simulink model "semifinal"  (R2020a)
settings: Solver=VariableStepAuto  StartTime=0.0  StopTime=50.0  RelTol=1e-3
undefined symbols (not defined in the file): D1, Delta
libraries: powerlib x39, sps_avr x2
settings Model: Creator=USER  LastModifiedBy=USER

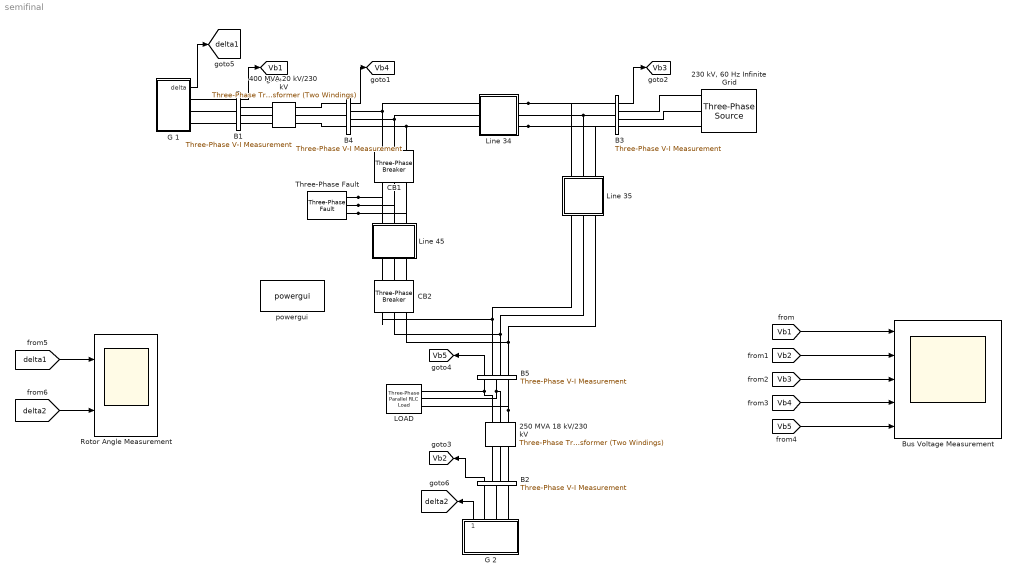
== system semifinal ==
  "    Line 35 " : Subsystem
  "230 kV, 60 Hz Infinite Grid" : powerlib/Electrical Sources/Three-Phase Source  InternalConnection=Yg  VoltagePhases=off  Voltage=230e3  PhaseAngle=0  Voltage_phases=[25e3 25e3 25e3]/sqrt(3)  PhaseAngles_phases=[0 -120 +120]  Frequency=60  NonIdealSource=on  SpecifyImpedance=off  Resistance=0.00000000000000001  Inductance=16.58e-3  ShortCircuitLevel=100e6  BaseVoltage=230e3  XRratio=7  BusType=swing  Pref=0  Qref=0  Prefabc=[10e3, 10e3, 10e3]  Qrefabc=[0, 0, 0]  Qmin=-inf  Qmax=inf
  250 MVA 18 kV/230 kV : powerlib/Elements/Three-Phase Transformer (Two Windings)  Winding1Connection=Delta (D1)  Winding2Connection=Yg  CoreType=Three single-phase transformers  SetSaturation=off  Hysteresis=off  DataFile='hysteresis'  SetInitialFlux=off  Measurements=None  UNITS=pu  NominalPower=[ 250e6 60 ]  Winding1="[ 18e3 0.002  0.0]"  Winding2=[ 230e3 0.002 0.04]  Rm=inf  Lm=inf  L0=0.5  Saturation="[ 0,0  ;  0.005,1.2  ;  1.0,1.4 ]"  InitialFluxes=[ 0.8 , -0.8 , 0.7 ]  BreakLoop=off  DiscreteSolver=Trapezoidal iterative  DataType=off  TransfoNumber=0
  400 MVA 20 kV/230 kV : powerlib/Elements/Three-Phase Transformer (Two Windings)  Winding1Connection=Delta (D1)  Winding2Connection=Yg  CoreType=Three single-phase transformers  SetSaturation=off  Hysteresis=off  DataFile='hysteresis'  SetInitialFlux=off  Measurements=None  UNITS=pu  NominalPower=[ 400E6 60 ]  Winding1="[ 20e3 0.002  0.0]"  Winding2=[ 230e3 0.002 0.022]  Rm=inf  Lm=inf  L0=0.5  Saturation="[ 0,0  ;  0.005,1.2  ;  1.0,1.4 ]"  InitialFluxes=[ 0.8 , -0.8 , 0.7 ]  BreakLoop=off  DiscreteSolver=Trapezoidal iterative  DataType=off  TransfoNumber=0
  B1 : powerlib/Measurements/Three-Phase V-I Measurement  VoltageMeasurement=phase-to-phase  SetLabelV=off  LabelV=Vabc_B1  Vpu=off  VpuLL=on  CurrentMeasurement=no  SetLabelI=off  LabelI=Iabc_B1  Ipu=off  Pbase=100e6  Vbase=20e3  OutputType=Magnitude  PhasorSimulation=on  PSBequivalent=0
  B2 : powerlib/Measurements/Three-Phase V-I Measurement  VoltageMeasurement=phase-to-phase  SetLabelV=off  LabelV=Vabc_B1  Vpu=off  VpuLL=on  CurrentMeasurement=no  SetLabelI=on  LabelI=Iabc_B1  Ipu=on  Pbase=100e6  Vbase=18e3  OutputType=Magnitude  PhasorSimulation=on  PSBequivalent=0
  B3 : powerlib/Measurements/Three-Phase V-I Measurement  VoltageMeasurement=phase-to-phase  SetLabelV=off  LabelV=Vabc_B1  Vpu=off  VpuLL=on  CurrentMeasurement=no  SetLabelI=off  LabelI=Iabc_B1  Ipu=on  Pbase=100e6  Vbase=230e3  OutputType=Magnitude  PhasorSimulation=on  PSBequivalent=0
  B4 : powerlib/Measurements/Three-Phase V-I Measurement  VoltageMeasurement=phase-to-phase  SetLabelV=off  LabelV=Vabc_B1  Vpu=off  VpuLL=on  CurrentMeasurement=no  SetLabelI=off  LabelI=Iabc_B1  Ipu=on  Pbase=100e6  Vbase=230e3  OutputType=Magnitude  PhasorSimulation=on  PSBequivalent=0
  B5 : powerlib/Measurements/Three-Phase V-I Measurement  VoltageMeasurement=phase-to-phase  SetLabelV=off  LabelV=Vabc_B1  Vpu=off  VpuLL=on  CurrentMeasurement=no  SetLabelI=on  LabelI=Iabc_B1  Ipu=on  Pbase=100e6  Vbase=230e3  OutputType=Magnitude  PhasorSimulation=on  PSBequivalent=0
  Bus Voltage Measurement : Scope  NumInputPorts=5
  CB1 : powerlib/Elements/Three-Phase Breaker  InitialState=closed  SwitchA=on  SwitchB=on  SwitchC=on  SwitchTimes=[20.3]  External=off  BreakerResistance=0.001  SnubberResistance=1e6  SnubberCapacitance=inf  Measurements=None
  CB2 : powerlib/Elements/Three-Phase Breaker  InitialState=closed  SwitchA=on  SwitchB=on  SwitchC=on  SwitchTimes=[20.3]  External=off  BreakerResistance=0.001  SnubberResistance=1e6  SnubberCapacitance=inf  Measurements=None
  G 1 : Subsystem
  G 2 : Subsystem
  "LOAD " : powerlib/Elements/Three-Phase Parallel RLC Load  LConnTagsString=A|B|C  Configuration=Y (grounded)  NominalVoltage=230e3  Vabc=[1e3 1e3 1e3]  Vabcp=[1e3 1e3 1e3]  NominalFrequency=60  UnbalancedPower=off  ActivePower=0.5e8  InductivePower=0.16e8  CapacitivePower=0  Pabc=[10e3 9e3 11e3]  QLabc=[100 90 110]  QCabc=[100 90 110]  Pabcp=[10e3 9e3 11e3]  QLabcp=[100 90 110]  QCabcp=[100 90 110]  Measurements=None  LoadType=constant Z
  Line 34 : Subsystem
  Line 45 : Subsystem
  Rotor Angle Measurement : Scope  NumInputPorts=2
  Three-Phase Fault : powerlib/Elements/Three-Phase Fault  InitialStates=0  FaultA=on  FaultB=on  FaultC=on  GroundFault=on  SwitchTimes=[20]  External=off  SwitchStatus=NaN  FaultResistance=0.001  GroundResistance=0.2  SnubberResistance=1e6  SnubberCapacitance=inf  Measurements=None
  powergui : powerlib/powergui  Priority=1  SimulationMode=Phasor  SampleTime=50e-6  frequency=60  Iterations=50  frequencyindice=60  Pbase=100e6  ErrMax=1e-4  UnitsV=kV  UnitsW=MW  buscounter=0  FunctionMessages=off  echomessages=off  EnableUseOfTLC=off  CurrentSourceSwitches=off  DisableSnubberDevices=off  DisableRonSwitches=off  DisableVfSwitches=off  DisplayEquations=off  AutomaticDiscreteSolvers=off  SolverType=Tustin/Backward Euler (TBE)  Interpol=off  ExternalGateDelay=off  methode=off  Ts=100  x0status=blocks  SPID=on  SwTol=0  HookPort=off  NonlinearTolerance=1e-4  nMaxIteration=100  ContinueOnMaxIteration=off  RestoreLinks=warning  ResistiveCurrentMeasurement=off  Frange=[0:2:500]  Ylog=off  Xlog=on  ShowGrid=off  save=off  variable=ZData  structure=0  ZoomFFT=off  StartTime=0.0  cycles=1  DisplayStyle=1  fundamental=60  FreqAxis=off  MaxFrequency=1000  frequencyindicesteady=1  RmsSteady=1  display=off
  tag scope: Vb1=global, Vb2=global, Vb3=global, Vb4=global, Vb5=global, delta1=global, delta2=global
  wires:
  B1/1 -> [Vb1]
  B4/1 -> [Vb4]
  G 1/1(delta) -> [delta1]
  B2/1 -> [Vb2]
  G 2/1(delta) -> [delta2]
  B5/1 -> [Vb5]
  B3/1 -> [Vb3]
  [delta1] -> Rotor Angle Measurement/1
  [delta2] -> Rotor Angle Measurement/2
  [Vb2] -> Bus Voltage Measurement/2
  [Vb3] -> Bus Voltage Measurement/3
  [Vb5] -> Bus Voltage Measurement/5
  [Vb4] -> Bus Voltage Measurement/4
  [Vb1] -> Bus Voltage Measurement/1
  connections:
  G 1/RConn3 -- B1/LConn3
  B1/LConn2 -- G 1/RConn2
  400 MVA 20 kV/230 kV/LConn1 -- B1/RConn1
  400 MVA 20 kV/230 kV/RConn2 -- B4/LConn2
  B1/RConn2 -- 400 MVA 20 kV/230 kV/LConn2
  B1/LConn1 -- G 1/RConn1
  400 MVA 20 kV/230 kV/RConn3 -- B4/LConn3
  400 MVA 20 kV/230 kV/RConn1 -- B4/LConn1
  400 MVA 20 kV/230 kV/LConn3 -- B1/RConn3
  B5/LConn2 -- "LOAD "/LConn2 -- 250 MVA 18 kV/230 kV/RConn2
  B5/LConn1 -- "LOAD "/LConn1 -- 250 MVA 18 kV/230 kV/RConn1
  250 MVA 18 kV/230 kV/RConn3 -- "LOAD "/LConn3 -- B5/LConn3
  B2/LConn2 -- G 2/RConn2
  B2/RConn1 -- 250 MVA 18 kV/230 kV/LConn1
  B2/LConn1 -- G 2/RConn1
  B2/RConn2 -- 250 MVA 18 kV/230 kV/LConn2
  B2/LConn3 -- G 2/RConn3
  B2/RConn3 -- 250 MVA 18 kV/230 kV/LConn3
  Three-Phase Fault/LConn3 -- Line 45/RConn3 -- CB1/RConn3
  Three-Phase Fault/LConn2 -- Line 45/RConn2 -- CB1/RConn2
  Three-Phase Fault/LConn1 -- CB1/RConn1 -- Line 45/RConn1
  CB2/LConn3 -- Line 45/LConn3
  CB2/LConn1 -- Line 45/LConn1
  CB2/LConn2 -- Line 45/LConn2
  Line 34/LConn1 -- "    Line 35 "/LConn1 -- B3/LConn1
  Line 34/LConn3 -- "    Line 35 "/LConn3 -- B3/LConn3
  "230 kV, 60 Hz Infinite Grid"/RConn1 -- B3/RConn1
  "230 kV, 60 Hz Infinite Grid"/RConn2 -- B3/RConn2
  "230 kV, 60 Hz Infinite Grid"/RConn3 -- B3/RConn3
  Line 34/RConn1 -- CB1/LConn1 -- B4/RConn1
  B4/RConn2 -- CB1/LConn2 -- Line 34/RConn2
  Line 34/RConn3 -- CB1/LConn3 -- B4/RConn3
  "    Line 35 "/RConn1 -- CB2/RConn1 -- B5/RConn1
  B5/RConn2 -- CB2/RConn2 -- "    Line 35 "/RConn2
  B5/RConn3 -- CB2/RConn3 -- "    Line 35 "/RConn3
  "    Line 35 "/LConn2 -- B3/LConn2 -- Line 34/LConn2

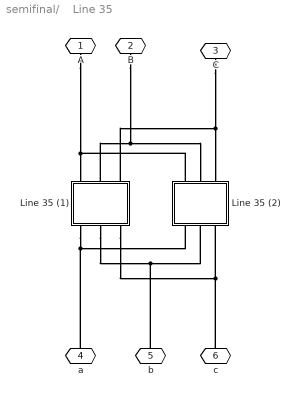
== system semifinal/    Line 35  ==
  Line 35 (1) : Subsystem
  Line 35 (2) : Subsystem
  A : PMIOPort  Side=Left
  B : PMIOPort  Port=2  Side=Left
  C : PMIOPort  Port=3  Side=Left
  a : PMIOPort  Port=4  Side=Right
  b : PMIOPort  Port=5  Side=Right
  c : PMIOPort  Port=6  Side=Right
  connections:
  A/RConn1 -- Line 35 (1)/LConn1 -- Line 35 (2)/LConn1
  Line 35 (1)/LConn2 -- Line 35 (2)/LConn2 -- B/RConn1
  Line 35 (1)/LConn3 -- Line 35 (2)/LConn3 -- C/RConn1
  Line 35 (1)/RConn1 -- Line 35 (2)/RConn1 -- a/RConn1
  Line 35 (1)/RConn2 -- Line 35 (2)/RConn2 -- b/RConn1
  Line 35 (1)/RConn3 -- Line 35 (2)/RConn3 -- c/RConn1

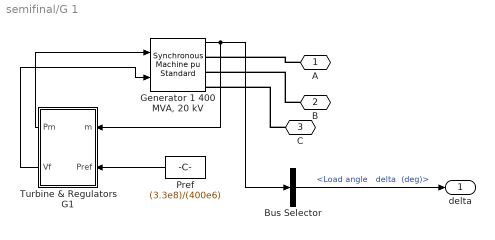
== system semifinal/G 1 ==
  Bus Selector : BusSelector  OutputSignals="Load angle   delta  (deg)"
  "Generator 1 400 MVA, 20 kV" : powerlib/Machines/Synchronous Machine pu Standard  PresetModel=No  MechanicalLoad=Mechanical power Pm  ShowDetailedParameters=on  RotorType=Salient-pole  Units=per unit standard parameters  MeasurementBus=off  NominalParameters="[400E6  20e3   60 ]"  Reactances1=[ 31 32 33 34 35 36 37 ]  Reactances2=[ 1.305, 0.067, 0.252, 0.474, 0.243, 0.18 ]  dAxisTimeConstants=Short-circuit  qAxisTimeConstants=Open-circuit  TimeConstants1=[]  TimeConstants2=[]  TimeConstants3=[]  TimeConstants4=[]  TimeConstants5=[ 1.01, 0.053, 0.1 ]  TimeConstants6=[]  TimeConstants7=[]  TimeConstants8=[]  StatorResistance=0  Mechanical="[ 11.2 0  32]"  PolePairs=32  InitialConditions=[0 -16.6861 0.950218 0.950218 0.950218 48.1093 -71.8907 168.109 1.44424]  SetSaturation=off  Saturation=[0.6404,0.7127,0.8441,0.9214,0.9956,1.082,1.19,1.316,1.457;0.7,0.7698,0.8872,0.9466,0.9969,1.046,1.1,1.151,1.201]  LoadFlowParameters=[1 950000000 0 0]  TsPowergui=0  TsBlock=-1  IterativeModel=Forward Euler  IterativeDiscreteModel=Trapezoidal non iterative  BusType=PV  Pref=3.3e8  Qref=0  Qmin=-Inf  Qmax=Inf  PLF=0  QLF=0
      settings: AttributesFormatString=\n\n
  Pref : Constant  Value=(3.3e8)/(400e6)
  Turbine & Regulators G1 : Subsystem
  A : PMIOPort  Side=Right
  B : PMIOPort  Port=2  Side=Right
  C : PMIOPort  Port=3  Side=Right
  delta : Outport
  wires:
  Turbine & Regulators G1/1(Pm) -> "Generator 1 400 MVA, 20 kV"/1
  Turbine & Regulators G1/2(Vf) -> "Generator 1 400 MVA, 20 kV"/2
  Pref/1 -> Turbine & Regulators G1/2(Pref)
  "Generator 1 400 MVA, 20 kV"/1 -> Turbine & Regulators G1/1(m), Bus Selector/1
  Bus Selector/1 -> delta/1  "<Load angle   delta  (deg)>"
  connections:
  A/RConn1 -- "Generator 1 400 MVA, 20 kV"/RConn1
  B/RConn1 -- "Generator 1 400 MVA, 20 kV"/RConn2
  C/RConn1 -- "Generator 1 400 MVA, 20 kV"/RConn3

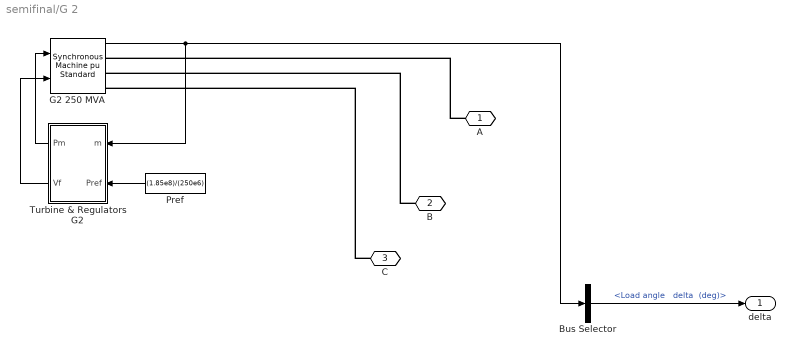
== system semifinal/G 2 ==
  Bus Selector : BusSelector  OutputSignals="Load angle   delta  (deg)"
  G2 250 MVA : powerlib/Machines/Synchronous Machine pu Standard  PresetModel=No  MechanicalLoad=Mechanical power Pm  ShowDetailedParameters=on  RotorType=Salient-pole  Units=per unit standard parameters  MeasurementBus=off  NominalParameters="[250E6  18e3   60 ]"  Reactances1=[ 31 32 33 34 35 36 37 ]  Reactances2=[ 1.305, 0.1, 0.252, 0.474, 0.243, 0.18 ]  dAxisTimeConstants=Short-circuit  qAxisTimeConstants=Open-circuit  TimeConstants1=[]  TimeConstants2=[]  TimeConstants3=[]  TimeConstants4=[]  TimeConstants5=[ 1.01, 0.053, 0.1 ]  TimeConstants6=[]  TimeConstants7=[]  TimeConstants8=[]  StatorResistance=2.8544e-3  Mechanical="[ 8 0  32]"  PolePairs=32  InitialConditions=[0 -69.7487 0.812764 0.812764 0.812764 -5.44703 -125.447 114.553 1.40021]  SetSaturation=off  Saturation=[0.6404,0.7127,0.8441,0.9214,0.9956,1.082,1.19,1.316,1.457;0.7,0.7698,0.8872,0.9466,0.9969,1.046,1.1,1.151,1.201]  LoadFlowParameters=[2 4000000000 0 0]  TsPowergui=0  TsBlock=-1  IterativeModel=Forward Euler  IterativeDiscreteModel=Trapezoidal non iterative  BusType=PV  Pref=1.85e8  Qref=0  Qmin=-Inf  Qmax=Inf  PLF=0  QLF=0
      settings: AttributesFormatString=\n\n
  Pref : Constant  Value=(1.85e8)/(250e6)
  Turbine & Regulators G2 : Subsystem
  A : PMIOPort  Side=Right
  B : PMIOPort  Port=2  Side=Right
  C : PMIOPort  Port=3  Side=Right
  delta : Outport
  wires:
  Pref/1 -> Turbine & Regulators G2/2(Pref)
  Turbine & Regulators G2/1(Pm) -> G2 250 MVA/1
  Turbine & Regulators G2/2(Vf) -> G2 250 MVA/2
  G2 250 MVA/1 -> Turbine & Regulators G2/1(m), Bus Selector/1
  Bus Selector/1 -> delta/1  "<Load angle   delta  (deg)>"
  connections:
  A/RConn1 -- G2 250 MVA/RConn1
  B/RConn1 -- G2 250 MVA/RConn2
  C/RConn1 -- G2 250 MVA/RConn3

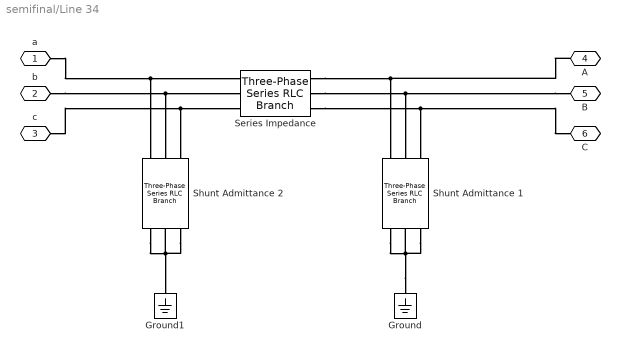
== system semifinal/Line 34 ==
  Ground : powerlib/Elements/Ground  LConnTagsString=a
  Ground1 : powerlib/Elements/Ground  LConnTagsString=a
  Series Impedance : powerlib/Elements/Three-Phase Series RLC Branch  LConnTagsString=A|B|C  RConnTagsString=A|B|C  BranchType=RL  Resistance=(((230e3)^2)/100e6)*0.007  Inductance=((((230e3)^2)/100e6)*0.040)/(2*pi*60)  Capacitance=1e-6  Measurements=None
  Shunt Admittance 1 : powerlib/Elements/Three-Phase Series RLC Branch  LConnTagsString=A|B|C  RConnTagsString=A|B|C  BranchType=C  Resistance=1.0  Inductance=1e-3  Capacitance=((((100e6/((230e3)^2))*0.082))/(2*pi*60))/2  Measurements=None
  Shunt Admittance 2 : powerlib/Elements/Three-Phase Series RLC Branch  LConnTagsString=A|B|C  RConnTagsString=A|B|C  BranchType=C  Resistance=1.0  Inductance=1e-3  Capacitance=((((100e6/((230e3)^2))*0.082))/(2*pi*60))/2  Measurements=None
  a : PMIOPort  Side=Right
  b : PMIOPort  Port=2  Side=Right
  c : PMIOPort  Port=3  Side=Right
  A : PMIOPort  Port=4  Side=Left
  B : PMIOPort  Port=5  Side=Left
  C : PMIOPort  Port=6  Side=Left
  connections:
  Ground/LConn1 -- Shunt Admittance 1/RConn3 -- Shunt Admittance 1/RConn2 -- Shunt Admittance 1/RConn1
  a/RConn1 -- Series Impedance/LConn1 -- Shunt Admittance 2/LConn1
  b/RConn1 -- Series Impedance/LConn2 -- Shunt Admittance 2/LConn2
  c/RConn1 -- Series Impedance/LConn3 -- Shunt Admittance 2/LConn3
  A/RConn1 -- Shunt Admittance 1/LConn1 -- Series Impedance/RConn1
  B/RConn1 -- Shunt Admittance 1/LConn2 -- Series Impedance/RConn2
  C/RConn1 -- Series Impedance/RConn3 -- Shunt Admittance 1/LConn3
  Shunt Admittance 2/RConn1 -- Shunt Admittance 2/RConn2 -- Shunt Admittance 2/RConn3 -- Ground1/LConn1

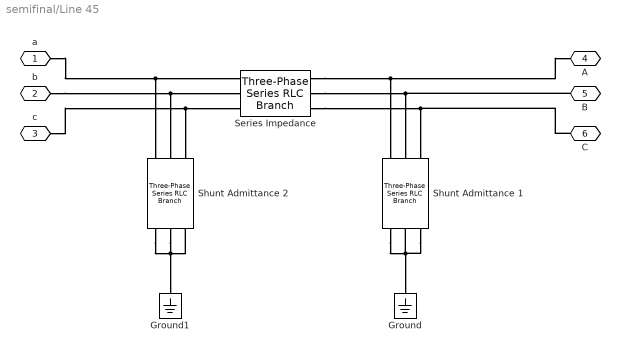
== system semifinal/Line 45 ==
  Ground : powerlib/Elements/Ground  LConnTagsString=a
  Ground1 : powerlib/Elements/Ground  LConnTagsString=a
  Series Impedance : powerlib/Elements/Three-Phase Series RLC Branch  LConnTagsString=A|B|C  RConnTagsString=A|B|C  BranchType=RL  Resistance=(((230e3)^2)/100e6)*0.018  Inductance=((((230e3)^2)/100e6)*0.110)/(2*pi*60)  Capacitance=1e-6  Measurements=None
  Shunt Admittance 1 : powerlib/Elements/Three-Phase Series RLC Branch  LConnTagsString=A|B|C  RConnTagsString=A|B|C  BranchType=C  Resistance=1  Inductance=1e-3  Capacitance=((((100e6/((230e3)^2))*0.226))/(2*pi*60))/2  Measurements=None
  Shunt Admittance 2 : powerlib/Elements/Three-Phase Series RLC Branch  LConnTagsString=A|B|C  RConnTagsString=A|B|C  BranchType=C  Resistance=1  Inductance=1e-3  Capacitance=((((100e6/((230e3)^2))*0.226))/(2*pi*60))/2  Measurements=None
  a : PMIOPort  Side=Right
  b : PMIOPort  Port=2  Side=Right
  c : PMIOPort  Port=3  Side=Right
  A : PMIOPort  Port=4  Side=Left
  B : PMIOPort  Port=5  Side=Left
  C : PMIOPort  Port=6  Side=Left
  connections:
  Shunt Admittance 1/RConn3 -- Shunt Admittance 1/RConn2 -- Ground/LConn1 -- Shunt Admittance 1/RConn1
  a/RConn1 -- Series Impedance/LConn1 -- Shunt Admittance 2/LConn1
  b/RConn1 -- Series Impedance/LConn2 -- Shunt Admittance 2/LConn2
  c/RConn1 -- Series Impedance/LConn3 -- Shunt Admittance 2/LConn3
  Series Impedance/RConn1 -- A/RConn1 -- Shunt Admittance 1/LConn1
  Series Impedance/RConn2 -- B/RConn1 -- Shunt Admittance 1/LConn2
  Series Impedance/RConn3 -- C/RConn1 -- Shunt Admittance 1/LConn3
  Shunt Admittance 2/RConn1 -- Shunt Admittance 2/RConn3 -- Shunt Admittance 2/RConn2 -- Ground1/LConn1

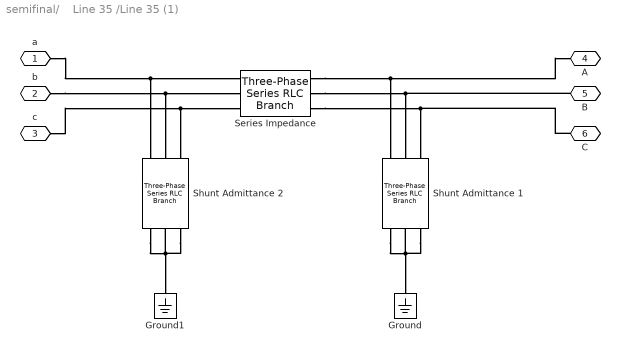
== system semifinal/    Line 35 /Line 35 (1) ==
  Ground : powerlib/Elements/Ground  LConnTagsString=a
  Ground1 : powerlib/Elements/Ground  LConnTagsString=a
  Series Impedance : powerlib/Elements/Three-Phase Series RLC Branch  LConnTagsString=A|B|C  RConnTagsString=A|B|C  BranchType=RL  Resistance=(((230e3)^2)/100e6)*0.008  Inductance=((((230e3)^2)/100e6)*0.047)/(2*pi*60)  Capacitance=1e-6  Measurements=None
  Shunt Admittance 1 : powerlib/Elements/Three-Phase Series RLC Branch  LConnTagsString=A|B|C  RConnTagsString=A|B|C  BranchType=C  Resistance=1  Inductance=1e-3  Capacitance=((((100e6/((230e3)^2))*0.098))/(2*pi*60))/2  Measurements=None
  Shunt Admittance 2 : powerlib/Elements/Three-Phase Series RLC Branch  LConnTagsString=A|B|C  RConnTagsString=A|B|C  BranchType=C  Resistance=1  Inductance=1e-3  Capacitance=((((100e6/((230e3)^2))*0.098))/(2*pi*60))/2  Measurements=None
  a : PMIOPort  Side=Right
  b : PMIOPort  Port=2  Side=Right
  c : PMIOPort  Port=3  Side=Right
  A : PMIOPort  Port=4  Side=Left
  B : PMIOPort  Port=5  Side=Left
  C : PMIOPort  Port=6  Side=Left
  connections:
  Shunt Admittance 1/RConn3 -- Shunt Admittance 1/RConn2 -- Ground/LConn1 -- Shunt Admittance 1/RConn1
  a/RConn1 -- Series Impedance/LConn1 -- Shunt Admittance 2/LConn1
  b/RConn1 -- Series Impedance/LConn2 -- Shunt Admittance 2/LConn2
  c/RConn1 -- Series Impedance/LConn3 -- Shunt Admittance 2/LConn3
  Series Impedance/RConn1 -- A/RConn1 -- Shunt Admittance 1/LConn1
  Series Impedance/RConn2 -- B/RConn1 -- Shunt Admittance 1/LConn2
  Series Impedance/RConn3 -- C/RConn1 -- Shunt Admittance 1/LConn3
  Shunt Admittance 2/RConn1 -- Shunt Admittance 2/RConn2 -- Shunt Admittance 2/RConn3 -- Ground1/LConn1

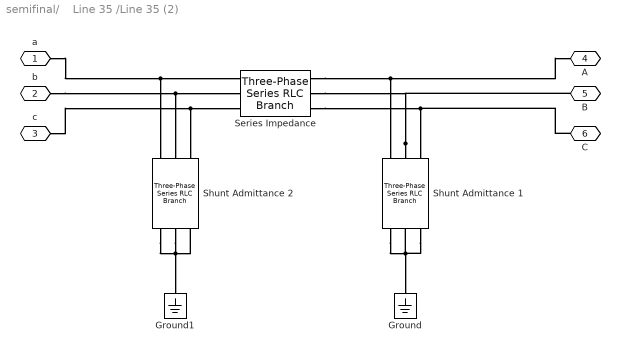
== system semifinal/    Line 35 /Line 35 (2) ==
  Ground : powerlib/Elements/Ground  LConnTagsString=a
  Ground1 : powerlib/Elements/Ground  LConnTagsString=a
  Series Impedance : powerlib/Elements/Three-Phase Series RLC Branch  LConnTagsString=A|B|C  RConnTagsString=A|B|C  BranchType=RL  Resistance=(((230e3)^2)/100e6)*0.008  Inductance=((((230e3)^2)/100e6)*0.047)/(2*pi*60)  Capacitance=1e-6  Measurements=None
  Shunt Admittance 1 : powerlib/Elements/Three-Phase Series RLC Branch  LConnTagsString=A|B|C  RConnTagsString=A|B|C  BranchType=C  Resistance=1  Inductance=1e-3  Capacitance=((((100e6/((230e3)^2))*0.098))/(2*pi*60))/2  Measurements=None
  Shunt Admittance 2 : powerlib/Elements/Three-Phase Series RLC Branch  LConnTagsString=A|B|C  RConnTagsString=A|B|C  BranchType=C  Resistance=1  Inductance=1e-3  Capacitance=((((100e6/((230e3)^2))*0.098))/(2*pi*60))/2  Measurements=None
  a : PMIOPort  Side=Right
  b : PMIOPort  Port=2  Side=Right
  c : PMIOPort  Port=3  Side=Right
  A : PMIOPort  Port=4  Side=Left
  B : PMIOPort  Port=5  Side=Left
  C : PMIOPort  Port=6  Side=Left
  connections:
  Shunt Admittance 1/RConn3 -- Shunt Admittance 1/RConn2 -- Ground/LConn1 -- Shunt Admittance 1/RConn1
  a/RConn1 -- Series Impedance/LConn1 -- Shunt Admittance 2/LConn1
  b/RConn1 -- Series Impedance/LConn2 -- Shunt Admittance 2/LConn2
  c/RConn1 -- Series Impedance/LConn3 -- Shunt Admittance 2/LConn3
  Series Impedance/RConn1 -- A/RConn1 -- Shunt Admittance 1/LConn1
  Shunt Admittance 1/LConn2 -- Series Impedance/RConn2 -- B/RConn1
  Series Impedance/RConn3 -- C/RConn1 -- Shunt Admittance 1/LConn3
  Shunt Admittance 2/RConn1 -- Shunt Admittance 2/RConn3 -- Shunt Admittance 2/RConn2 -- Ground1/LConn1

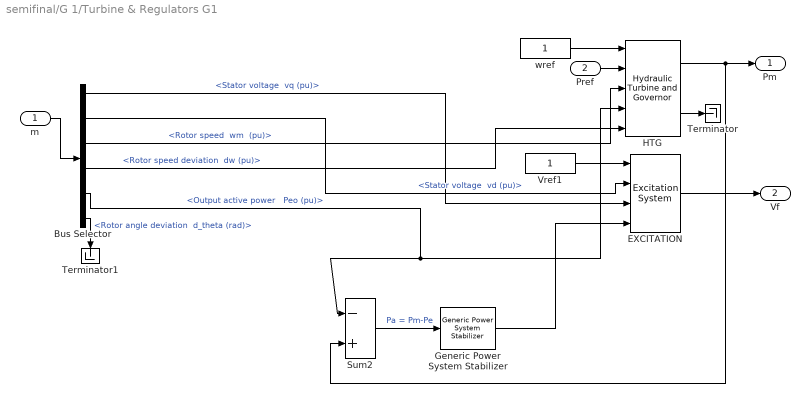
== system semifinal/G 1/Turbine & Regulators G1 ==
  m : Inport
  Pref : Inport  Port=2
  Bus Selector : BusSelector  OutputSignals="dq0 components.Stator voltage  vq (pu),dq0 components.Stator voltage  vd (pu),Mechanical.Rotor speed  wm  (pu),Mechanical.Rotor speed deviation  dw (pu),Output active power   Peo (pu),Mechanical.Rotor angle deviation  d_theta (rad)"
  EXCITATION : sps_avr/Excitation System  tr=20e-3  reg=[ 50, 0.001 ]  exc=[ 1, 0 ]  tgr=[ 0, 0 ]  damp=[ 0.001, 0.1 ]  sat=[ 0, 0 ]  lim="[ 0,  7, 0 ]"  v0=[1,1]
      settings: SourceProductBaseCode=PS
  Generic Power System Stabilizer : powerlib/Machines/Generic Power System Stabilizer  Tsensor=15e-3  K=2  Twashout=0.7  Tleadlag1="[60e-3  0.5]"  Tleadlag2=[0 0]  VSlimits=[-0.15 0.15]  Vinit=0  Plot_On=off  MagdB_On=on  FreqRange=logspace(-2,2,500)
      settings: SourceProductBaseCode=PS
  HTG : powerlib/Machines/Hydraulic Turbine and Governor  sm="[ 10/3  0.07 ]"  gate="[  0.01  0.97518  -0.1  0.1 ]"  reg="[  0.05  1.163  0.105  0  0.01  ]"  hyd="[  0  2.67  ]"  dref=0  po=1
      settings: SourceProductBaseCode=PS
  Sum2 : Sum  Inputs=-+  InputSameDT=on  SaturateOnIntegerOverflow=on  OutDataTypeStr=Inherit: Same as first input
  Terminator : Terminator
  Terminator1 : Terminator
  Vref1 : Constant
  wref : Constant
  Pm : Outport  InitialOutput=0
  Vf : Outport  Port=2  InitialOutput=0
  wires:
  HTG/2 -> Terminator/1
  Vref1/1 -> EXCITATION/1
  Pref/1 -> HTG/2
  wref/1 -> HTG/1
  HTG/1 -> Pm/1, Sum2/2
  EXCITATION/1 -> Vf/1
  Sum2/1 -> Generic Power System Stabilizer/1  "Pa = Pm-Pe"
  Generic Power System Stabilizer/1 -> EXCITATION/4
  m/1 -> Bus Selector/1
  Bus Selector/1 -> EXCITATION/3  "<Stator voltage  vq (pu)>"
  Bus Selector/2 -> EXCITATION/2  "<Stator voltage  vd (pu)>"
  Bus Selector/6 -> Terminator1/1  "<Rotor angle deviation  d_theta (rad)>"
  Bus Selector/3 -> HTG/3  "<Rotor speed  wm  (pu)>"
  Bus Selector/4 -> HTG/5  "<Rotor speed deviation  dw (pu)>"
  Bus Selector/5 -> Sum2/1, HTG/4  "<Output active power   Peo (pu)>"

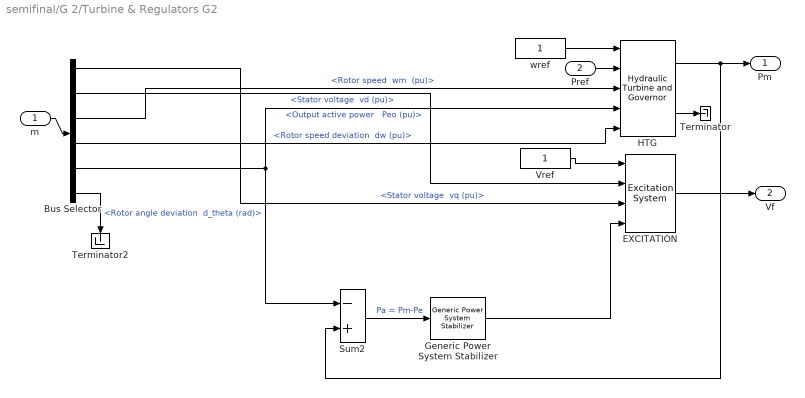
== system semifinal/G 2/Turbine & Regulators G2 ==
  m : Inport
  Pref : Inport  Port=2
  Bus Selector : BusSelector  OutputSignals="dq0 components.Stator voltage  vq (pu),dq0 components.Stator voltage  vd (pu),Mechanical.Rotor speed  wm  (pu),Mechanical.Rotor speed deviation  dw (pu),Output active power   Peo (pu),Mechanical.Rotor angle deviation  d_theta (rad)"
  EXCITATION : sps_avr/Excitation System  tr=20e-3  reg=[ 50, 0.001 ]  exc=[ 1, 0 ]  tgr=[ 0, 0 ]  damp=[ 0.001, 0.1 ]  sat=[ 0, 0 ]  lim="[ 0,  7, 0 ]"  v0=[1,1]
      settings: SourceProductBaseCode=PS
  Generic Power System Stabilizer : powerlib/Machines/Generic Power System Stabilizer  Tsensor=15e-3  K=2  Twashout=0.7  Tleadlag1="[60e-3  0.5]"  Tleadlag2=[0 0]  VSlimits=[-0.15 0.15]  Vinit=0  Plot_On=off  MagdB_On=on  FreqRange=logspace(-2,2,500)
      settings: SourceProductBaseCode=PS
  HTG : powerlib/Machines/Hydraulic Turbine and Governor  sm="[ 10/3  0.07 ]"  gate="[  0.01  0.97518  -0.1  0.1 ]"  reg="[  0.05  1.163  0.105  0  0.01  ]"  hyd="[  0  2.67  ]"  dref=0  po=1
      settings: SourceProductBaseCode=PS
  Sum2 : Sum  Inputs=-+  InputSameDT=on  SaturateOnIntegerOverflow=on  OutDataTypeStr=Inherit: Same as first input
  Terminator : Terminator
  Terminator2 : Terminator
  Vref : Constant
  wref : Constant
  Pm : Outport  InitialOutput=0
  Vf : Outport  Port=2  InitialOutput=0
  wires:
  EXCITATION/1 -> Vf/1
  HTG/1 -> Sum2/2, Pm/1
  wref/1 -> HTG/1
  Pref/1 -> HTG/2
  Vref/1 -> EXCITATION/1
  HTG/2 -> Terminator/1
  Generic Power System Stabilizer/1 -> EXCITATION/4
  Sum2/1 -> Generic Power System Stabilizer/1  "Pa = Pm-Pe"
  Bus Selector/6 -> Terminator2/1  "<Rotor angle deviation  d_theta (rad)>"
  Bus Selector/1 -> EXCITATION/3  "<Stator voltage  vq (pu)>"
  Bus Selector/2 -> EXCITATION/2  "<Stator voltage  vd (pu)>"
  Bus Selector/3 -> HTG/3  "<Rotor speed  wm  (pu)>"
  Bus Selector/4 -> HTG/5  "<Rotor speed deviation  dw (pu)>"
  Bus Selector/5 -> HTG/4, Sum2/1  "<Output active power   Peo (pu)>"
  m/1 -> Bus Selector/1
